simulink model "robot3_model_slidingmode_control_step"  (R2023b)
settings: Solver=ode3  StartTime=0.0  StopTime=2*pi  RelTol=1e-3
undefined symbols (not defined in the file): Coriolis3, Dhat3, Dinv3, Forward_kin3, Gravity3
libraries: simulink x1
settings Model: Creator=사용자  LastModifiedBy=사용자
settings SolverCC: ZeroCrossAlgorithm=Adaptive
settings DebuggingCC: IgnoredZcDiagnostic=none

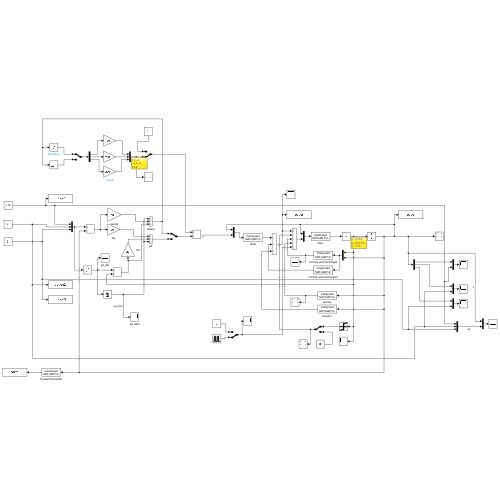
[thumbnail: Simulink's stored preview of the top-level diagram]
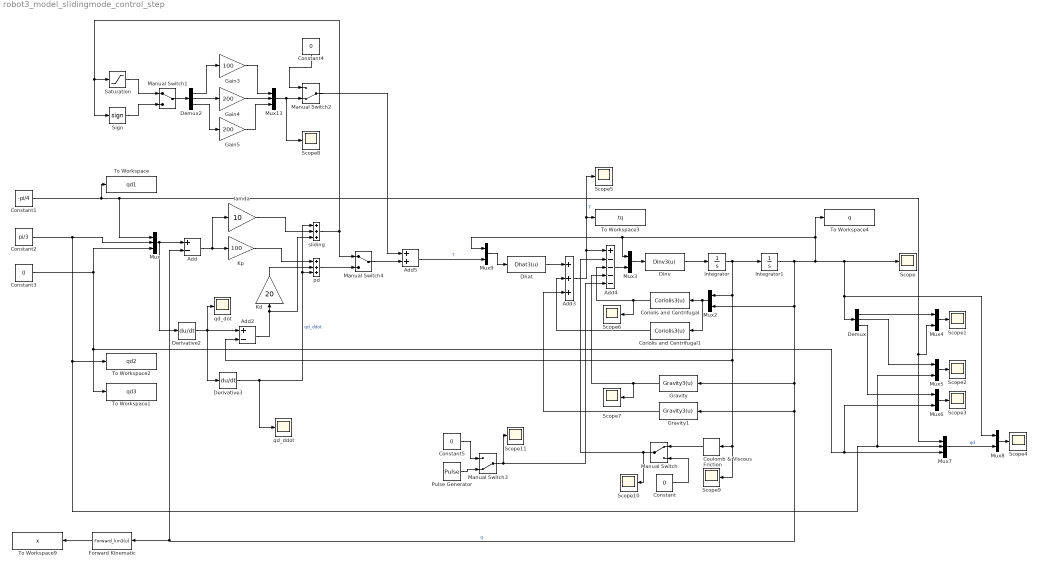
== system robot3_model_slidingmode_control_step ==
  Add : Sum  Inputs=+-
  Add2 : Sum  Inputs=+-
  Add3 : Sum  Inputs=+++
  Add4 : Sum  Inputs=+----
  Add5 : Sum
  Constant : Constant  Value=0
  Constant1 : Constant  Value=-pi/4  SampleTime=0.001
  Constant2 : Constant  Value=pi/3  SampleTime=0.001
  Constant3 : Constant  Value=0  SampleTime=0.001
  Constant4 : Constant  Value=0
  Constant5 : Constant  Value=0
  Coriolis and Centrifugal : MATLABFcn  MATLABFcn=Coriolis3(u)  OutputDimensions=3  Output1D=off
  Coriolis and Centrifugal1 : MATLABFcn  MATLABFcn=Coriolis3(u)  OutputDimensions=3  Output1D=off
  Coulomb & Viscous Friction : simulink/Discontinuities/Coulomb & Viscous Friction  offset=10  gain=5
  Demux : Demux  Outputs=3
  Demux2 : Demux  Outputs=3
  Derivative2 : Derivative
  Derivative3 : Derivative
  Dhat : MATLABFcn  MATLABFcn=Dhat3(u)  OutputDimensions=3  Output1D=off
  Dinv : MATLABFcn  MATLABFcn=Dinv3(u)  OutputDimensions=3  Output1D=off
  Forward Kinematic : MATLABFcn  MATLABFcn=Forward_kin3(u)  OutputDimensions=3  Output1D=off
  Gain3 : Gain  Gain=100
  Gain4 : Gain  Gain=200
  Gain5 : Gain  Gain=200
  Gravity : MATLABFcn  MATLABFcn=Gravity3(u)  OutputDimensions=3  Output1D=off
  Gravity1 : MATLABFcn  MATLABFcn=Gravity3(u)  OutputDimensions=3  Output1D=off
  Integrator : Integrator  InitialCondition=[0;0;0];
  Integrator1 : Integrator  InitialCondition=[0;pi/2;-pi/2]
  Kd : Gain  Gain=20
  Kp : Gain  Gain=100
  Manual Switch : ManualSwitch
  Manual Switch1 : ManualSwitch
  Manual Switch2 : ManualSwitch  CurrentSetting=0
  Manual Switch3 : ManualSwitch  CurrentSetting=0
  Manual Switch4 : ManualSwitch
  Mux : Mux  Inputs=3
  Mux13 : Mux  Inputs=3
  Mux{2..6,8..9} (7 alike) : Mux  Inputs=2
  Mux7 : Mux  Inputs=3
  Pulse Generator : DiscretePulseGenerator  PulseType=Time based  Amplitude=100  PulseWidth=2  PhaseDelay=2
  Saturation : Saturate  UpperLimit=1  LowerLimit=-1  ZeroCross=off
  Scope{,1..11} (12 alike) : Scope
  Sign : Signum  ZeroCross=off
  To Workspace : ToWorkspace  VariableName=qd1  SaveFormat=Timeseries  SampleTime=0.001
  To Workspace1 : ToWorkspace  VariableName=qd3  SaveFormat=Timeseries  SampleTime=0.001
  To Workspace2 : ToWorkspace  VariableName=qd2  SaveFormat=Timeseries  SampleTime=0.001
  To Workspace3 : ToWorkspace  VariableName=tq  SaveFormat=Timeseries  SampleTime=0.001
  To Workspace4 : ToWorkspace  VariableName=q  SaveFormat=Timeseries  SampleTime=0.001
  To Workspace9 : ToWorkspace  VariableName=x  SampleTime=0.001
  lamda : Gain  Gain=10
  pd : Sum  Inputs=+++
  qd_ddot : Scope
  qd_dot : Scope
  sliding : Sum  Inputs=+++
  wires:
  Mux/1 -> Add/1, Derivative2/1
  Constant3/1 -> Mux/3, To Workspace1/1, Mux6/2, Mux7/3
  Add2/1 -> sliding/3, Kd/1
  Kp/1 -> pd/1
  Kd/1 -> pd/2
  Add/1 -> lamda/1, Kp/1
  Dinv/1 -> Integrator/1
  Mux2/1 -> Coriolis and Centrifugal/1, Coriolis and Centrifugal1/1
  Integrator/1 -> Scope9/1, Coulomb & Viscous Friction/1, Add2/2, Mux2/1, Integrator1/1
  Integrator1/1 -> Mux2/2, Forward Kinematic/1, Add/2, Gravity1/1, Gravity/1, Demux/1, Mux8/1, Scope/1, Mux3/1, Mux9/1, To Workspace4/1  "q"
  Mux4/1 -> Scope1/1
  Mux5/1 -> Scope2/1
  Mux6/1 -> Scope3/1
  Demux/1 -> Mux4/1
  Demux/2 -> Mux5/1
  Demux/3 -> Mux6/1
  Constant1/1 -> Mux7/1, Mux4/2, Mux/1, To Workspace/1
  Constant2/1 -> Mux5/2, Mux7/2, To Workspace2/1, Mux/2
  Mux7/1 -> Mux8/2  "qd"
  Mux8/1 -> Scope4/1
  Derivative3/1 -> qd_ddot/1, sliding/1, pd/3  "qd_ddot"
  Mux9/1 -> Dhat/1
  Mux3/1 -> Dinv/1
  Add4/1 -> Mux3/2
  Dhat/1 -> Add3/1
  Coriolis and Centrifugal1/1 -> Add3/2
  Gravity1/1 -> Add3/3
  Coriolis and Centrifugal/1 -> Scope6/1, Add4/3
  Gravity/1 -> Scope7/1, Add4/4
  Add3/1 -> Scope5/1, To Workspace3/1, Add4/1  "T"
  Constant/1 -> Manual Switch/2
  Manual Switch/1 -> Scope10/1, Add4/2
  Coulomb & Viscous Friction/1 -> Manual Switch/1
  Derivative2/1 -> qd_dot/1, Derivative3/1, Add2/1
  Demux2/3 -> Gain5/1
  Manual Switch2/1 -> Add5/1
  sliding/1 -> Sign/1, Saturation/1, Manual Switch4/1
  Constant4/1 -> Manual Switch2/1
  Saturation/1 -> Manual Switch1/1
  Gain3/1 -> Mux13/1
  Gain5/1 -> Mux13/3
  Manual Switch1/1 -> Demux2/1
  Mux13/1 -> Scope8/1, Manual Switch2/2
  Demux2/1 -> Gain3/1
  Sign/1 -> Manual Switch1/2
  Demux2/2 -> Gain4/1
  Gain4/1 -> Mux13/2
  Pulse Generator/1 -> Manual Switch3/2
  Constant5/1 -> Manual Switch3/1
  Manual Switch3/1 -> Scope11/1, Add4/5
  Add5/1 -> Mux9/2  "T"
  Manual Switch4/1 -> Add5/2
  pd/1 -> Manual Switch4/2
  lamda/1 -> sliding/2
  Forward Kinematic/1 -> To Workspace9/1
